simulink model "elvator_motion"  (R2014a)
settings: Solver=ode45  StartTime=0.0  StopTime=10.0  RelTol=1e-3
settings Model: Creator=Rishabh  LastModifiedBy=Rishabh

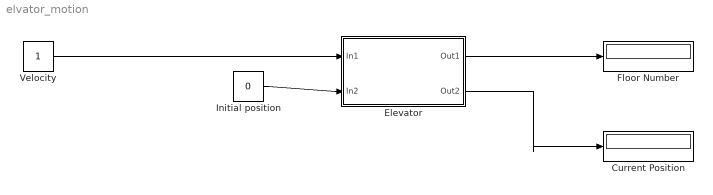
== system elvator_motion ==
  Current Position : Display
  Elevator : Subsystem
  Floor Number : Display
  Initial position : Constant  Value=0
  Velocity : Constant
  wires:
  Velocity/1 -> Elevator/1(In1)
  Initial position/1 -> Elevator/2(In2)
  Elevator/1(Out1) -> Floor Number/1
  Elevator/2(Out2) -> Current Position/1

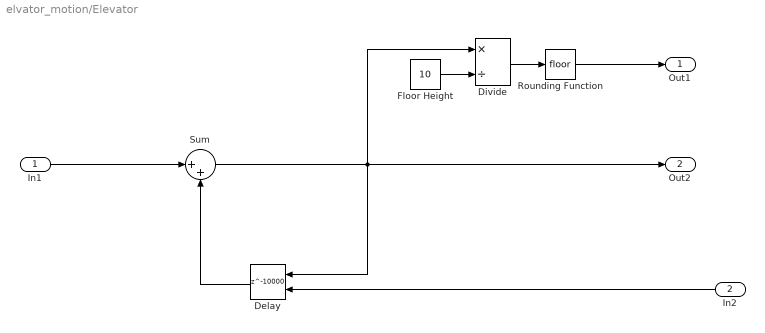
== system elvator_motion/Elevator ==
  In1 : Inport
  In2 : Inport  Port=2
  Delay : Delay  DelayLength=10000  InitialConditionSource=Input port  InitialCondition=2  SampleTime=.00001
      settings: InputPortMap=u0,p4
  Divide : Product  Inputs=*/  RndMeth=Nearest  LockScale=on
  Floor Height : Constant  Value=10
  Rounding Function : Rounding
  Sum : Sum  Inputs=|++
  Out1 : Outport
  Out2 : Outport  Port=2
  wires:
  Delay/1 -> Sum/2
  In1/1 -> Sum/1
  Sum/1 -> Out2/1, Divide/1, Delay/1
  In2/1 -> Delay/2
  Divide/1 -> Rounding Function/1
  Floor Height/1 -> Divide/2
  Rounding Function/1 -> Out1/1
